simulink model "integ_verify_prove"  (R2014b)
settings: Solver=FixedStepDiscrete  StartTime=0.0  StopTime=10.0  FixedStep=0.01  RelTol=1e-3
undefined symbols (not defined in the file): sldvsubsys
libraries: simulink x16, sldvlib x14
settings Model: Creator=Natasha  LastModifiedBy=JYOGANAN
settings DebuggingCC: UnderspecifiedInitializationDetection=Classic  MergeDetectMultiDrivingBlocksExec=none
settings ConfigComp: Description=Design Verifier Custom Configuration Component  DVMode=PropertyProving  DVMaxTestCaseSteps=500  DVTestSuiteOptimization=CombinedObjectives (Nonlinear Extended)  DVDetectActiveLogic=on

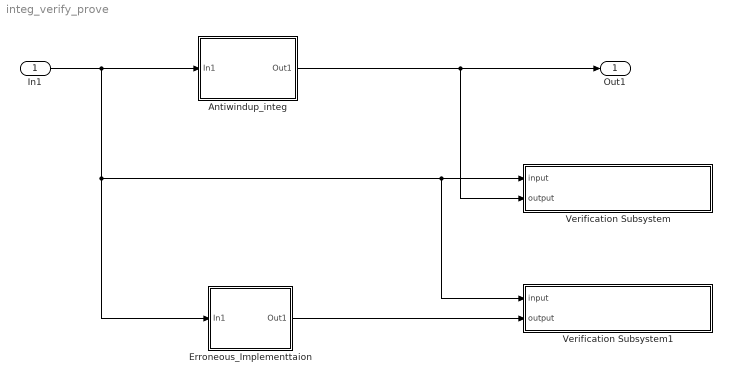
== system integ_verify_prove ==
  In1 : Inport
  Antiwindup_integ : Subsystem
  Erroneous_Implementtaion : Subsystem
  Verification Subsystem : Subsystem  Tag=VerificationSubsystem  DisableCoverage=on  LoadFcn=sldvsubsys('check')  TreatAsAtomicUnit=on  SimViewingDevice=on  mask(VerificationSubsystem){}
      mask init:
      | sldvsubsys('maskInit');
      settings: CopyFcn=sldvsubsys('copy');  OpenFcn=open_system(gcb,'force');
      settings: PreSaveFcn=|
      | set_param(gcb,'SimViewingDevice','on');
      | sldvsubsys('check');
      mask Help: helpview(fullfile(docroot,'toolbox','sldv','sldv.map'),'verificationsubsystem')
      mask Display: image(imread('sldvicon_versubsys.png','BackGroundColor',[1 1 1]),'center');
  Verification Subsystem1 : Subsystem  Tag=VerificationSubsystem  DisableCoverage=on  LoadFcn=sldvsubsys('check')  TreatAsAtomicUnit=on  SimViewingDevice=on  mask(VerificationSubsystem){}
      mask init:
      | sldvsubsys('maskInit');
      settings: CopyFcn=sldvsubsys('copy');  OpenFcn=open_system(gcb,'force');
      settings: PreSaveFcn=|
      | set_param(gcb,'SimViewingDevice','on');
      | sldvsubsys('check');
      mask Help: helpview(fullfile(docroot,'toolbox','sldv','sldv.map'),'verificationsubsystem')
      mask Display: image(imread('sldvicon_versubsys.png','BackGroundColor',[1 1 1]),'center');
  Out1 : Outport
  wires:
  In1/1 -> Verification Subsystem1/1(input), Verification Subsystem/1(input), Erroneous_Implementtaion/1(In1), Antiwindup_integ/1(In1)
  Antiwindup_integ/1(Out1) -> Out1/1, Verification Subsystem/2(output)
  Erroneous_Implementtaion/1(Out1) -> Verification Subsystem1/2(output)

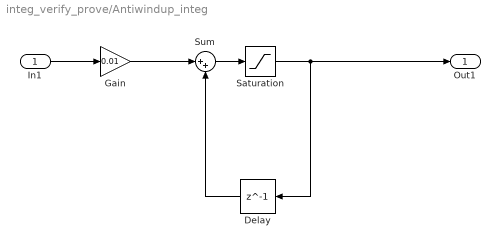
== system integ_verify_prove/Antiwindup_integ ==
  In1 : Inport
  Delay : Delay  DelayLength=1  InitialCondition=0
  Gain : Gain  Gain=0.01
  Saturation : Saturate
  Sum : Sum  Inputs=|++
  Out1 : Outport
  wires:
  Sum/1 -> Saturation/1
  Gain/1 -> Sum/1
  Saturation/1 -> Out1/1, Delay/1
  Delay/1 -> Sum/2
  In1/1 -> Gain/1

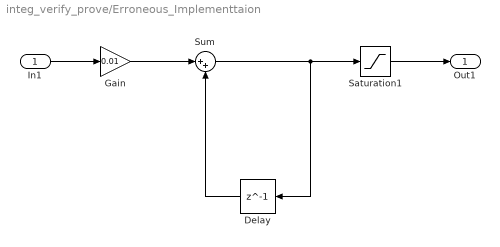
== system integ_verify_prove/Erroneous_Implementtaion ==
  In1 : Inport
  Delay : Delay  DelayLength=1  InitialCondition=0
  Gain : Gain  Gain=0.01
  Saturation1 : Saturate
  Sum : Sum  Inputs=|++
  Out1 : Outport
  wires:
  In1/1 -> Gain/1
  Delay/1 -> Sum/2
  Gain/1 -> Sum/1
  Sum/1 -> Saturation1/1, Delay/1
  Saturation1/1 -> Out1/1

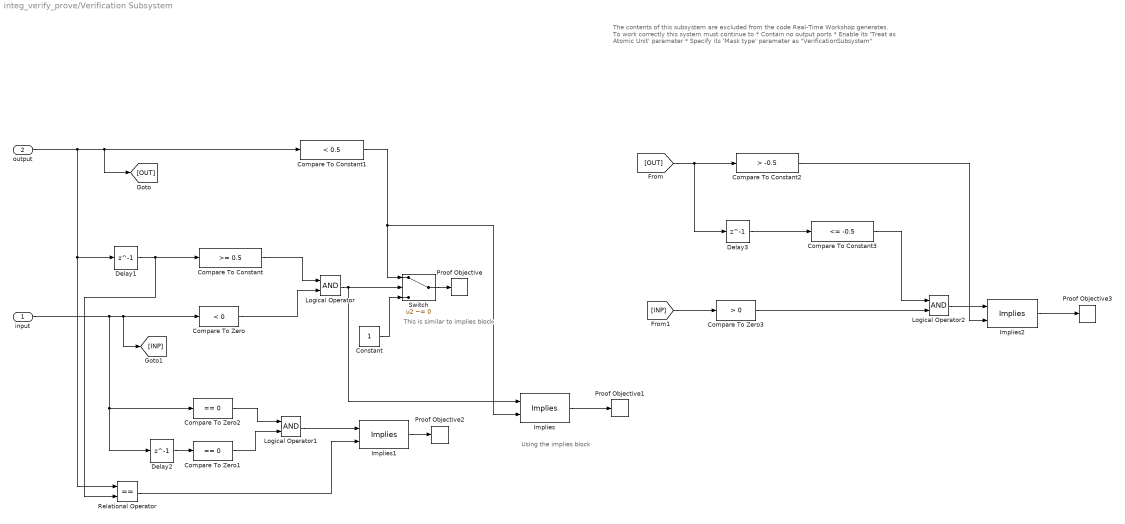
== system integ_verify_prove/Verification Subsystem ==
  note: Using the implies block
  note: This is similar to
      | implies block
  note: The contents of this subsystem are excluded from the code Real-Time
      | Workshop generates.
      |
      | To work correctly this system must continue to
      | * Contain no output ports
      | * Enable its 'Treat as Atomic Unit' parameter
      | * Specify its 'Mask type' parameter as "VerificationSubsystem"
  input : Inport
  output : Inport  Port=2
  Compare To Constant : simulink/Logic and Bit Operations/Compare To Constant  relop=>=  const=0.5  OutDataTypeStr=boolean
  Compare To Constant1 : simulink/Logic and Bit Operations/Compare To Constant  relop=<  const=0.5  OutDataTypeStr=boolean
  Compare To Constant2 : simulink/Logic and Bit Operations/Compare To Constant  relop=>  const=-0.5  OutDataTypeStr=boolean
  Compare To Constant3 : simulink/Logic and Bit Operations/Compare To Constant  relop=<=  const=-0.5  OutDataTypeStr=boolean
  Compare To Zero : simulink/Logic and Bit Operations/Compare To Zero  relop=<  OutDataTypeStr=boolean
  Compare To Zero1 : simulink/Logic and Bit Operations/Compare To Zero  relop===  OutDataTypeStr=boolean
  Compare To Zero2 : simulink/Logic and Bit Operations/Compare To Zero  relop===  OutDataTypeStr=boolean
  Compare To Zero3 : simulink/Logic and Bit Operations/Compare To Zero  relop=>  OutDataTypeStr=boolean
  Constant : Constant
  Delay1 : Delay  DelayLength=1  InitialCondition=0
  Delay2 : Delay  DelayLength=1  InitialCondition=0
  Delay3 : Delay  DelayLength=1  InitialCondition=0
  Implies : sldvlib/Verification Utilities/Implies
  Implies1 : sldvlib/Verification Utilities/Implies
  Implies2 : sldvlib/Verification Utilities/Implies
  Logical Operator : Logic  AllPortsSameDT=off  OutDataTypeStr=boolean
  Logical Operator1 : Logic  AllPortsSameDT=off  OutDataTypeStr=boolean
  Logical Operator2 : Logic  AllPortsSameDT=off  OutDataTypeStr=boolean
  Proof Objective{,1..3} (4 alike) : sldvlib/Objectives and Constraints/Proof Objective  enabled=on  customAVTBlockType=Proof Objective  intervals=1  dispValues=on  outEnabled=off  enableStopSim=off
      settings: AttributesFormatString=%<intervals>
  Relational Operator : RelationalOperator  Operator===  OutDataTypeStr=boolean
  Switch : Switch  Criteria=u2 ~= 0
  wires:
  input/1 -> Compare To Zero2/1, Delay2/1, [INP], Compare To Zero/1
  Compare To Constant/1 -> Logical Operator/1
  Compare To Zero/1 -> Logical Operator/2
  Logical Operator/1 -> Implies/1, Switch/2
  Constant/1 -> Switch/3
  Switch/1 -> Proof Objective/1
  output/1 -> [OUT], Compare To Constant1/1, Relational Operator/1, Delay1/1
  Compare To Constant1/1 -> Switch/1, Implies/2
  Implies/1 -> Proof Objective1/1
  Delay2/1 -> Compare To Zero1/1
  Compare To Zero2/1 -> Logical Operator1/1
  Compare To Zero1/1 -> Logical Operator1/2
  Logical Operator1/1 -> Implies1/1
  Delay1/1 -> Relational Operator/2, Compare To Constant/1
  Relational Operator/1 -> Implies1/2
  Implies1/1 -> Proof Objective2/1
  [OUT] -> Delay3/1, Compare To Constant2/1
  Delay3/1 -> Compare To Constant3/1
  [INP] -> Compare To Zero3/1
  Compare To Constant3/1 -> Logical Operator2/1
  Compare To Zero3/1 -> Logical Operator2/2
  Logical Operator2/1 -> Implies2/1
  Compare To Constant2/1 -> Implies2/2
  Implies2/1 -> Proof Objective3/1

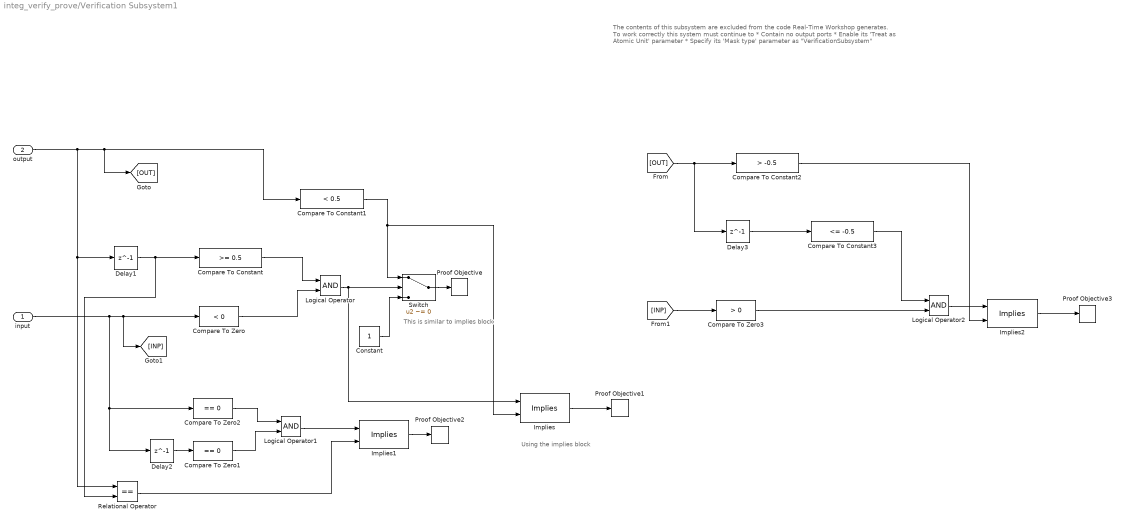
== system integ_verify_prove/Verification Subsystem1 ==
  note: The contents of this subsystem are excluded from the code Real-Time
      | Workshop generates.
      |
      | To work correctly this system must continue to
      | * Contain no output ports
      | * Enable its 'Treat as Atomic Unit' parameter
      | * Specify its 'Mask type' parameter as "VerificationSubsystem"
  note: This is similar to
      | implies block
  note: Using the implies block
  input : Inport
  output : Inport  Port=2
  Compare To Constant : simulink/Logic and Bit Operations/Compare To Constant  relop=>=  const=0.5  OutDataTypeStr=boolean
  Compare To Constant1 : simulink/Logic and Bit Operations/Compare To Constant  relop=<  const=0.5  OutDataTypeStr=boolean
  Compare To Constant2 : simulink/Logic and Bit Operations/Compare To Constant  relop=>  const=-0.5  OutDataTypeStr=boolean
  Compare To Constant3 : simulink/Logic and Bit Operations/Compare To Constant  relop=<=  const=-0.5  OutDataTypeStr=boolean
  Compare To Zero : simulink/Logic and Bit Operations/Compare To Zero  relop=<  OutDataTypeStr=boolean
  Compare To Zero1 : simulink/Logic and Bit Operations/Compare To Zero  relop===  OutDataTypeStr=boolean
  Compare To Zero2 : simulink/Logic and Bit Operations/Compare To Zero  relop===  OutDataTypeStr=boolean
  Compare To Zero3 : simulink/Logic and Bit Operations/Compare To Zero  relop=>  OutDataTypeStr=boolean
  Constant : Constant
  Delay1 : Delay  DelayLength=1  InitialCondition=0
  Delay2 : Delay  DelayLength=1  InitialCondition=0
  Delay3 : Delay  DelayLength=1  InitialCondition=0
  Implies : sldvlib/Verification Utilities/Implies
  Implies1 : sldvlib/Verification Utilities/Implies
  Implies2 : sldvlib/Verification Utilities/Implies
  Logical Operator : Logic  AllPortsSameDT=off  OutDataTypeStr=boolean
  Logical Operator1 : Logic  AllPortsSameDT=off  OutDataTypeStr=boolean
  Logical Operator2 : Logic  AllPortsSameDT=off  OutDataTypeStr=boolean
  Proof Objective{,1..3} (4 alike) : sldvlib/Objectives and Constraints/Proof Objective  enabled=on  customAVTBlockType=Proof Objective  intervals=1  dispValues=on  outEnabled=off  enableStopSim=off
      settings: AttributesFormatString=%<intervals>
  Relational Operator : RelationalOperator  Operator===  OutDataTypeStr=boolean
  Switch : Switch  Criteria=u2 ~= 0
  wires:
  Implies2/1 -> Proof Objective3/1
  Compare To Constant2/1 -> Implies2/2
  Logical Operator2/1 -> Implies2/1
  Compare To Zero3/1 -> Logical Operator2/2
  Compare To Constant3/1 -> Logical Operator2/1
  [INP] -> Compare To Zero3/1
  Delay3/1 -> Compare To Constant3/1
  [OUT] -> Compare To Constant2/1, Delay3/1
  Implies1/1 -> Proof Objective2/1
  Relational Operator/1 -> Implies1/2
  Delay1/1 -> Compare To Constant/1, Relational Operator/2
  Logical Operator1/1 -> Implies1/1
  Compare To Zero1/1 -> Logical Operator1/2
  Compare To Zero2/1 -> Logical Operator1/1
  Delay2/1 -> Compare To Zero1/1
  Implies/1 -> Proof Objective1/1
  Compare To Constant1/1 -> Implies/2, Switch/1
  output/1 -> Delay1/1, Relational Operator/1, Compare To Constant1/1, [OUT]
  Switch/1 -> Proof Objective/1
  Constant/1 -> Switch/3
  Logical Operator/1 -> Switch/2, Implies/1
  Compare To Zero/1 -> Logical Operator/2
  Compare To Constant/1 -> Logical Operator/1
  input/1 -> Compare To Zero/1, [INP], Delay2/1, Compare To Zero2/1
